simulink model "SVPWM"  (R2020b)
settings: Solver=VariableStepAuto  StartTime=0.0  StopTime=1  RelTol=1e-3
libraries: simulink x12, powerlib_meascontrol x1, powerlib x1
settings Model: Creator=marcu  LastModifiedBy=1

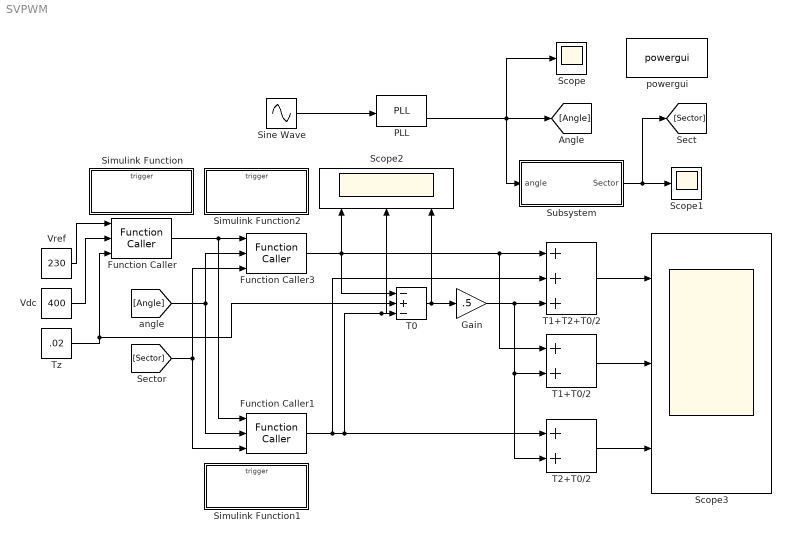
== system SVPWM ==
  Function Caller : FunctionCaller  FunctionPrototype=y = f1(u1,u2,u3)  InputArgumentSpecifications=<Enter example>  OutputArgumentSpecifications=<Enter example>
  Function Caller1 : FunctionCaller  FunctionPrototype=y = f2(u1,u2,u3)  InputArgumentSpecifications=<Enter example>  OutputArgumentSpecifications=<Enter example>
  Function Caller3 : FunctionCaller  FunctionPrototype=y = f3(u1,u2,u3)  InputArgumentSpecifications=<Enter example>  OutputArgumentSpecifications=<Enter example>
  Gain : Gain  Gain=.5
  PLL : powerlib_meascontrol/PLL/PLL  Fmin=45  Par_Init=[0, 60]  ParK=[180, 3200, 1]  TcD=1e-5  MaxRateChangeFreq=12  FilterCutOffFreq=25  Ts=1e-5  AGC=on
      settings: SourceProductBaseCode=PS
  Scope : Scope
  Scope1 : Scope
  Scope2 : Scope  NumInputPorts=3
  Scope3 : Scope  NumInputPorts=3
  Simulink Function : Subsystem  TreatAsAtomicUnit=on
  Simulink Function1 : Subsystem  TreatAsAtomicUnit=on
  Simulink Function2 : Subsystem  TreatAsAtomicUnit=on
  Sine Wave : Sin  Frequency=2*pi*50  SampleTime=0
  Subsystem : Subsystem
  T0 : Sum  Inputs=-+-
  T1+T0/2 : Sum
  T1+T2+T0/2 : Sum  Inputs=+++
  T2+T0/2 : Sum
  Tz : Constant  Value=.02
  Vdc : Constant  Value=400
  Vref : Constant  Value=230
  powergui : powerlib/powergui  Priority=1  SimulationMode=Continuous  SampleTime=50e-6  frequency=60  Iterations=50  frequencyindice=60  Pbase=100e6  ErrMax=1e-4  UnitsV=kV  UnitsW=MW  buscounter=0  FunctionMessages=off  echomessages=off  EnableUseOfTLC=off  CurrentSourceSwitches=off  DisableSnubberDevices=off  DisableRonSwitches=off  DisableVfSwitches=off  DisplayEquations=off  AutomaticDiscreteSolvers=off  SolverType=Tustin/Backward Euler (TBE)  Interpol=off  ExternalGateDelay=off  methode=off  Ts=100  x0status=blocks  SPID=on  SwTol=0  HookPort=off  NonlinearTolerance=1e-4  nMaxIteration=100  ContinueOnMaxIteration=off  RestoreLinks=warning  ResistiveCurrentMeasurement=off  Frange=[0:2:500]  Ylog=off  Xlog=on  ShowGrid=off  save=off  variable=ZData  structure=0  ZoomFFT=off  StartTime=0.0  cycles=1  DisplayStyle=1  fundamental=60  FreqAxis=off  MaxFrequency=1000  frequencyindicesteady=1  RmsSteady=1  display=off
  wires:
  Vdc/1 -> Function Caller/2
  Tz/1 -> Function Caller/3, T0/2
  Sine Wave/1 -> PLL/1
  PLL/2 -> Scope/1, [Angle], Subsystem/1(angle)
  Subsystem/1(Sector) -> [Sector], Scope1/1
  Function Caller/1 -> Function Caller1/1, Function Caller3/1
  [Angle] -> Function Caller1/2, Function Caller3/2
  [Sector] -> Function Caller1/3, Function Caller3/3
  Function Caller3/1 -> T0/1, T1+T0/2/1, T1+T2+T0/2/1, Scope2/1
  Function Caller1/1 -> T1+T2+T0/2/2, T0/3, Scope2/2, T2+T0/2/1
  T0/1 -> Gain/1, Scope2/3
  Vref/1 -> Function Caller/1
  Gain/1 -> T2+T0/2/2, T1+T0/2/2, T1+T2+T0/2/3
  T1+T0/2/1 -> Scope3/2
  T1+T2+T0/2/1 -> Scope3/1
  T2+T0/2/1 -> Scope3/3

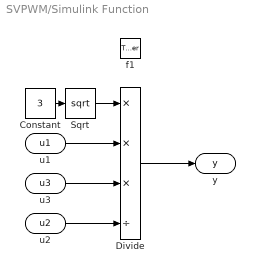
== system SVPWM/Simulink Function ==
  f1 : TriggerPort  TriggerType=function-call  IsSimulinkFunction=on  FunctionName=f1  FunctionVisibility=scoped  VariantControl=(inherit)
  Constant : Constant  Value=3
  Divide : Product  Inputs=***/
  Sqrt : Sqrt  SaturateOnIntegerOverflow=on
  u1 : ArgIn  DisableCoverage=on  ArgumentName=u1
  u2 : ArgIn  DisableCoverage=on  Port=2  ArgumentName=u2
  u3 : ArgIn  DisableCoverage=on  Port=3  ArgumentName=u3
  y : ArgOut  DisableCoverage=on  ArgumentName=y
  wires:
  u1/1 -> Divide/2
  u3/1 -> Divide/3
  u2/1 -> Divide/4
  Divide/1 -> y/1
  Sqrt/1 -> Divide/1
  Constant/1 -> Sqrt/1

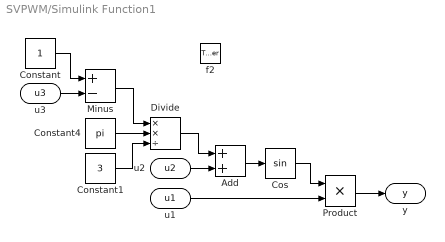
== system SVPWM/Simulink Function1 ==
  f2 : TriggerPort  TriggerType=function-call  IsSimulinkFunction=on  FunctionName=f2  FunctionVisibility=scoped  VariantControl=(inherit)
  Add : Sum
  Constant : Constant
  Constant1 : Constant  Value=3
  Constant4 : Constant  Value=pi
  Cos : Trigonometry  NumberOfIterations=100
  Divide : Product  Inputs=**/
  Minus : Sum  Inputs=+-
  Product : Product
  u1 : ArgIn  DisableCoverage=on  ArgumentName=u1
  u2 : ArgIn  DisableCoverage=on  Port=2  ArgumentName=u2
  u3 : ArgIn  DisableCoverage=on  Port=3  ArgumentName=u3
  y : ArgOut  DisableCoverage=on  ArgumentName=y
  wires:
  u2/1 -> Add/2
  Product/1 -> y/1
  Cos/1 -> Product/1
  Divide/1 -> Add/1
  Add/1 -> Cos/1
  u1/1 -> Product/2
  Constant1/1 -> Divide/3
  Constant4/1 -> Divide/2
  Minus/1 -> Divide/1
  u3/1 -> Minus/2
  Constant/1 -> Minus/1

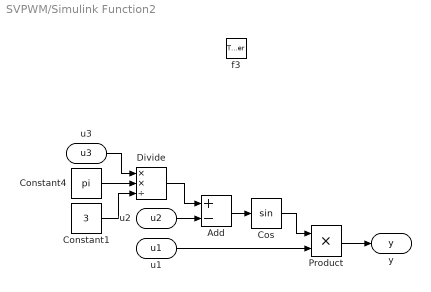
== system SVPWM/Simulink Function2 ==
  f3 : TriggerPort  TriggerType=function-call  IsSimulinkFunction=on  FunctionName=f3  FunctionVisibility=scoped  VariantControl=(inherit)
  Add : Sum  Inputs=+-
  Constant1 : Constant  Value=3
  Constant4 : Constant  Value=pi
  Cos : Trigonometry  NumberOfIterations=100
  Divide : Product  Inputs=**/
  Product : Product
  u1 : ArgIn  DisableCoverage=on  ArgumentName=u1
  u2 : ArgIn  DisableCoverage=on  Port=2  ArgumentName=u2
  u3 : ArgIn  DisableCoverage=on  Port=3  ArgumentName=u3
  y : ArgOut  DisableCoverage=on  ArgumentName=y
  wires:
  Add/1 -> Cos/1
  Cos/1 -> Product/1
  Product/1 -> y/1
  Divide/1 -> Add/1
  u1/1 -> Product/2
  u3/1 -> Divide/1
  Constant4/1 -> Divide/2
  Constant1/1 -> Divide/3
  u2/1 -> Add/2

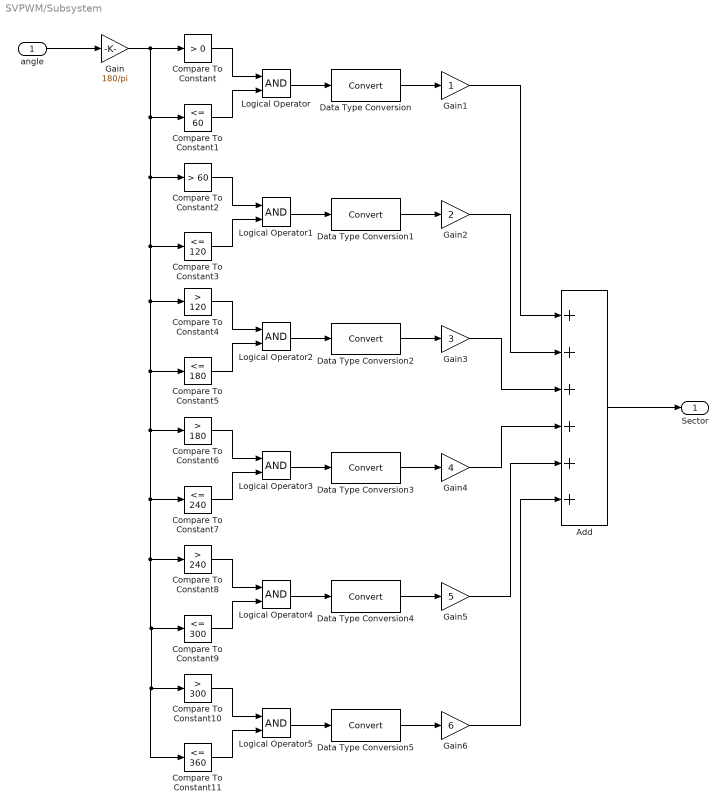
== system SVPWM/Subsystem ==
  angle : Inport
  Add : Sum  Inputs=++++++
  Compare To Constant : simulink/Logic and Bit Operations/Compare To Constant  relop=>  const=0  OutDataTypeStr=boolean
  Compare To Constant1 : simulink/Logic and Bit Operations/Compare To Constant  relop=<=  const=60  OutDataTypeStr=boolean
  Compare To Constant10 : simulink/Logic and Bit Operations/Compare To Constant  relop=>  const=300  OutDataTypeStr=boolean
  Compare To Constant11 : simulink/Logic and Bit Operations/Compare To Constant  relop=<=  const=360  OutDataTypeStr=boolean
  Compare To Constant2 : simulink/Logic and Bit Operations/Compare To Constant  relop=>  const=60  OutDataTypeStr=boolean
  Compare To Constant3 : simulink/Logic and Bit Operations/Compare To Constant  relop=<=  const=120  OutDataTypeStr=boolean
  Compare To Constant4 : simulink/Logic and Bit Operations/Compare To Constant  relop=>  const=120  OutDataTypeStr=boolean
  Compare To Constant5 : simulink/Logic and Bit Operations/Compare To Constant  relop=<=  const=180  OutDataTypeStr=boolean
  Compare To Constant6 : simulink/Logic and Bit Operations/Compare To Constant  relop=>  const=180  OutDataTypeStr=boolean
  Compare To Constant7 : simulink/Logic and Bit Operations/Compare To Constant  relop=<=  const=240  OutDataTypeStr=boolean
  Compare To Constant8 : simulink/Logic and Bit Operations/Compare To Constant  relop=>  const=240  OutDataTypeStr=boolean
  Compare To Constant9 : simulink/Logic and Bit Operations/Compare To Constant  relop=<=  const=300  OutDataTypeStr=boolean
  Data Type Conversion{,1..5} (6 alike) : DataTypeConversion
  Gain : Gain  Gain=180/pi
  Gain1 : Gain
  Gain2 : Gain  Gain=2
  Gain3 : Gain  Gain=3
  Gain4 : Gain  Gain=4
  Gain5 : Gain  Gain=5
  Gain6 : Gain  Gain=6
  Logical Operator{,1..5} (6 alike) : Logic  AllPortsSameDT=off  OutDataTypeStr=boolean
  Sector : Outport
  wires:
  angle/1 -> Gain/1
  Compare To Constant/1 -> Logical Operator/1
  Compare To Constant1/1 -> Logical Operator/2
  Logical Operator/1 -> Data Type Conversion/1
  Data Type Conversion/1 -> Gain1/1
  Data Type Conversion1/1 -> Gain2/1
  Logical Operator1/1 -> Data Type Conversion1/1
  Compare To Constant3/1 -> Logical Operator1/2
  Compare To Constant2/1 -> Logical Operator1/1
  Compare To Constant4/1 -> Logical Operator2/1
  Compare To Constant5/1 -> Logical Operator2/2
  Logical Operator2/1 -> Data Type Conversion2/1
  Data Type Conversion2/1 -> Gain3/1
  Data Type Conversion3/1 -> Gain4/1
  Logical Operator3/1 -> Data Type Conversion3/1
  Compare To Constant7/1 -> Logical Operator3/2
  Compare To Constant6/1 -> Logical Operator3/1
  Gain/1 -> Compare To Constant2/1, Compare To Constant7/1, Compare To Constant8/1, Compare To Constant11/1, Compare To Constant10/1, Compare To Constant9/1, Compare To Constant6/1, Compare To Constant5/1, Compare To Constant4/1, Compare To Constant3/1, Compare To Constant1/1, Compare To Constant/1
  Compare To Constant10/1 -> Logical Operator5/1
  Compare To Constant11/1 -> Logical Operator5/2
  Logical Operator5/1 -> Data Type Conversion5/1
  Data Type Conversion5/1 -> Gain6/1
  Data Type Conversion4/1 -> Gain5/1
  Logical Operator4/1 -> Data Type Conversion4/1
  Compare To Constant9/1 -> Logical Operator4/2
  Compare To Constant8/1 -> Logical Operator4/1
  Gain1/1 -> Add/1
  Gain2/1 -> Add/2
  Gain3/1 -> Add/3
  Gain4/1 -> Add/4
  Gain5/1 -> Add/5
  Gain6/1 -> Add/6
  Add/1 -> Sector/1
